simulink model "LQR"  (R2023b)
settings: Solver=VariableStepAuto  StartTime=0.0  StopTime=500.0  RelTol=1e-3
values from neighbouring files (symbols this model uses):
  A = double(A)    [consistent.m]    (also in dyn_model.m)
  B = double(B)    [consistent.m]    (also in dyn_model.m; rot_pend.m = [a b)
  ss_gain = 1/dcgain(cl_lq)    [consistent.m]
  x1_bar = 0    [consistent.m]    (also in dyn_model.m)
  x3_bar = pi    (= 3.14159265359)    [consistent.m]    (also in dyn_model.m = 0)
undefined symbols (not defined in the file or in its folder): K_lq
libraries: simulink_extras x5
settings Model: Creator=Mark  LastModifiedBy=Mark

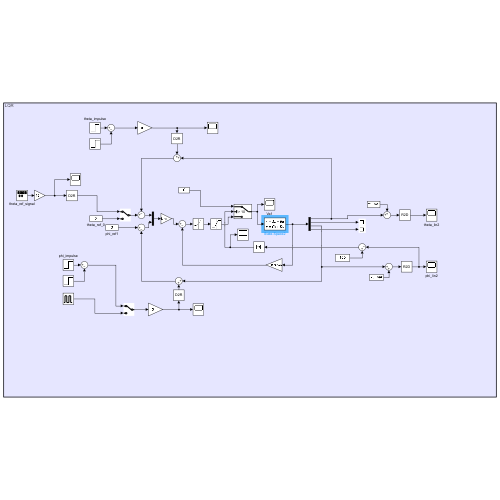
[thumbnail: Simulink's stored preview of the top-level diagram]
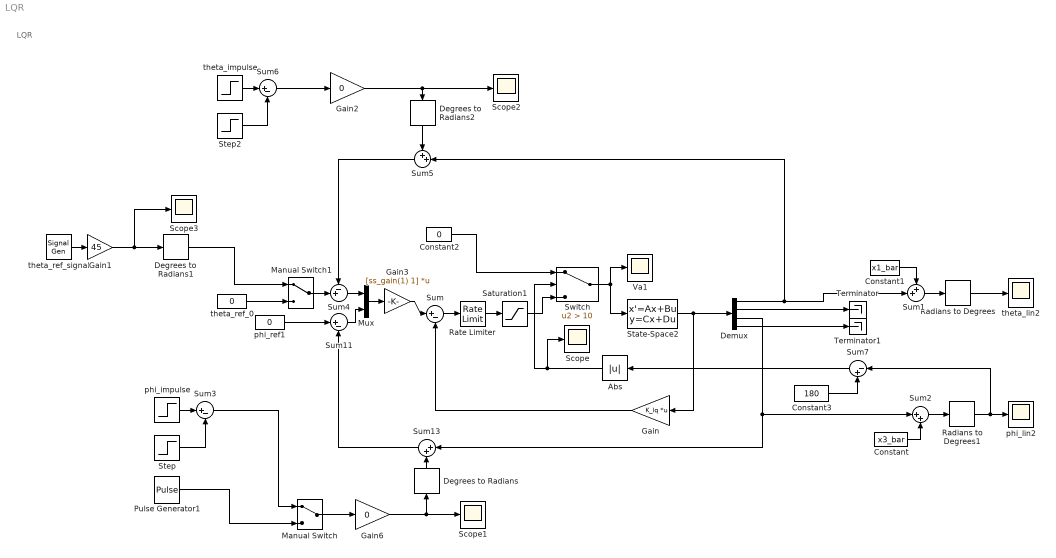
== system LQR ==
  note: LQR
  Abs : Abs  SaturateOnIntegerOverflow=off
  Constant : Constant  Value=x3_bar
  Constant1 : Constant  Value=x1_bar
  Constant2 : Constant  Value=0
  Constant3 : Constant  Value=180
  Degrees to Radians : simulink_extras/Transformations/Degrees to Radians
  Degrees to Radians1 : simulink_extras/Transformations/Degrees to Radians
  Degrees to Radians2 : simulink_extras/Transformations/Degrees to Radians
  Demux : Demux
  Gain : Gain  Gain=K_lq  Multiplication=Matrix(K*u) (u vector)
  Gain1 : Gain  Gain=45
  Gain2 : Gain  Gain=0
  Gain3 : Gain  Gain=[ss_gain(1) 1]  Multiplication=Matrix(K*u)
  Gain6 : Gain  Gain=0
  Manual Switch : ManualSwitch
  Manual Switch1 : ManualSwitch
  Mux : Mux  Inputs=2
  Pulse Generator1 : DiscretePulseGenerator  PulseType=Time based  Period=4  PulseWidth=50  PhaseDelay=10
  Radians to Degrees : simulink_extras/Transformations/Radians to Degrees
  Radians to Degrees1 : simulink_extras/Transformations/Radians to Degrees
  Rate Limiter : RateLimiter  RisingSlewLimit=inf  FallingSlewLimit=-inf  SampleTimeMode=inherited
  Saturation1 : Saturate  UpperLimit=10  LowerLimit=-10
  Scope{,1..3} (4 alike) : Scope
  State-Space2 : StateSpace  A=A  B=B  C=eye(4)  D=zeros(4,1)  InitialCondition=[0 0 0 0]
  Step : Step  Time=31  SampleTime=0
  Step2 : Step  Time=30.05  After=0  SampleTime=0
  Sum{,3,6,11} (4 alike) : Sum  Inputs=|+-
  Sum1 : Sum  Inputs=++|
  Sum13 : Sum  Inputs=|++
  Sum2 : Sum  Inputs=|++
  Sum4 : Sum  Inputs=-+|
  Sum5 : Sum  Inputs=++|
  Sum7 : Sum  Inputs=|-+
  Switch : Switch  Criteria=u2 > Threshold  Threshold=10  SaturateOnIntegerOverflow=off  InputSameDT=off
  Terminator : Terminator
  Terminator1 : Terminator
  Va1 : Scope
  phi_impulse : Step  Time=30  SampleTime=0
  phi_lin2 : Scope
  phi_ref1 : Constant  Value=0
  theta_impulse : Step  Time=30  SampleTime=0
  theta_lin2 : Scope
  theta_ref_0 : Constant  Value=0
  theta_ref_signal : SignalGenerator  Frequency=0.005
  wires:
  Degrees to Radians/1 -> Sum13/2
  Constant/1 -> Sum2/2
  Sum13/1 -> Sum11/2
  Sum1/1 -> Radians to Degrees/1
  Radians to Degrees1/1 -> Sum7/1, phi_lin2/1
  phi_ref1/1 -> Sum11/1
  Switch/1 -> State-Space2/1, Va1/1
  Demux/1 -> Sum5/2, Sum1/2
  Constant1/1 -> Sum1/1
  Sum2/1 -> Radians to Degrees1/1
  Demux/3 -> Sum2/1, Sum13/1
  Gain/1 -> Sum/2
  Rate Limiter/1 -> Saturation1/1
  Gain6/1 -> Scope1/1, Degrees to Radians/1
  State-Space2/1 -> Gain/1, Demux/1
  Radians to Degrees/1 -> theta_lin2/1
  Manual Switch/1 -> Gain6/1
  Sum/1 -> Rate Limiter/1
  Sum11/1 -> Mux/2
  Step/1 -> Sum3/2
  phi_impulse/1 -> Sum3/1
  Sum3/1 -> Manual Switch/1
  theta_ref_signal/1 -> Gain1/1
  Pulse Generator1/1 -> Manual Switch/2
  Sum4/1 -> Mux/1
  Gain1/1 -> Scope3/1, Degrees to Radians1/1
  Degrees to Radians1/1 -> Manual Switch1/1
  Gain2/1 -> Scope2/1, Degrees to Radians2/1
  Sum5/1 -> Sum4/1
  Degrees to Radians2/1 -> Sum5/1
  Sum6/1 -> Gain2/1
  Step2/1 -> Sum6/2
  theta_impulse/1 -> Sum6/1
  Manual Switch1/1 -> Sum4/2
  theta_ref_0/1 -> Manual Switch1/2
  Saturation1/1 -> Switch/3
  Constant2/1 -> Switch/1
  Abs/1 -> Scope/1, Switch/2
  Sum7/1 -> Abs/1
  Constant3/1 -> Sum7/2
  Gain3/1 -> Sum/1
  Mux/1 -> Gain3/1
  Demux/2 -> Terminator/1
  Demux/4 -> Terminator1/1
